simulink library "myLibrary"  (R2023b)
settings: Solver=VariableStepAuto  StartTime=0.0  StopTime=10.0  RelTol=1e-3
undefined symbols (not defined in the file): Cac_n1, ctrl1, Da, delta_slk, Discrete, dtha, ee_sli_rtmsupport, FA, gcbh, Ha, Ini, init_DCline, init_IPC, init_line, init_load, init_SG, init_shunt, init_TH, init_trafo, init_user, init_VSC, initMachineBlocks, Ka, Lf, Llkd_pu, Llkq1_pu, magnitude, NET, P, plots_step, q0, Rac_n1, Radd, Rkd_pu, Rkq1_pu, Rload_add, sim_config, sps_rtmsupport, spsSteamTurbineModel, T_DC_NET, T_global, T_IPC, T_load, T_NET, T_SG, T_shunt, T_STATCOM, T_TH, T_trafo, T_user, T_VSC, Ts, tstep, Udiff_a, V1
libraries: spsSeriesRLCBranchLib x120, eeGeneralControl x83, $bdroot x78, spsCurrentMeasurementLib x53, spsParallelRLCBranchLib x39, spsVoltageMeasurementLib x37, spsControlledVoltageSourceLib x30, simulink x29, spsFirstOrderFilterLib x18, spsMeasurementModel x13, spsThreePhaseVIMeasurementLib x5, dspsigops x4
(part 4 of 16)

== system myLibrary/SG_step ==
  Add : Sum  Inputs=-+
  Add1 : Sum
  Add2 : Sum  Inputs=+-
  Bus Selector : BusSelector  OutputSignals="Mechanical.Electromagnetic torque  Te (pu),dq0 components.Stator current  iq (pu),dq0 components.Stator current  id (pu),dq0 components.Field current  ifd (pu),dq0 components.Damper winding current  ikd (pu),dq0 components.Damper winding current  ikq1 (pu),dq0 components.Damper winding current  ikq2 (pu),dq0 components.Stator voltage  vq (pu),dq0 components.Stator voltage  vd (pu),Mechanical.Rotor angle deviation  d_theta (rad),Mechanical.Rotor speed  wm (pu),Mechanical.Rotor mechanical angle  theta (deg),Load angle   delta  (deg)"
  Constant4 : Constant  Value=[2/3 1/3; -1/3 1/3 ; -1/3 -2/3]
  Constant_pi1 : Constant  Value=pi/2
  Constant_pi2 : Constant  Value=-pi/2
  Current Measurement3 : spsCurrentMeasurementLib/Current Measurement  PhasorSimulation=off  OutputType=Complex  PSBequivalent=0
  Demux4 : Demux  Outputs=3
  Display : Display
  Display1 : Display
  Exciter : Subsystem
  Gain : Gain  Gain=T_SG.wb
  Gain1 : Gain  Gain=pi/180
  Gain2 : Gain  Gain=1/T_SG.Lmd_pu
  Gain3 : Gain  Gain=pi/180
  Governor-Turbine : Subsystem
  Integrator : Integrator
  Mux4 : Mux  Inputs=2
  PLL (3ph) : spsPLL3phLib/PLL (3ph)  Fmin=45  Par_Init=[0, 50]  ParK=[180, 3200, 1]  TcD=1e-4  MaxRateChangeFreq=12  FilterCutOffFreq=25  Ts=0  AGC=on
  PLL (3ph)1 : spsPLL3phLib/PLL (3ph)  Fmin=45  Par_Init=[initSG.theta_in, 50]  ParK=[180, 3200, 1]  TcD=1e-4  MaxRateChangeFreq=12  FilterCutOffFreq=25  Ts=0  AGC=on
  Pm : Step  Time=tstep_P  Before=initSG.Pm  After=initSG.Pm*(1+sim_config.DR)  SampleTime=1e-4
  SM1 : spsSynchronousMachinepuFundamentalLib/Synchronous Machine pu Fundamental  PresetModel=No  MechanicalLoad=Mechanical power Pm  ShowDetailedParameters=on  RotorType=Round  Units=per unit fundamental parameters  MeasurementBus=off  NominalParameters=initMachineBlocks{SGnum,1}  Stator=initMachineBlocks{SGnum,2}  Field=initMachineBlocks{SGnum,3}  Dampers2=initMachineBlocks{SGnum,4}  Dampers1="[ Rkd_pu   Llkd_pu  Rkq1_pu  Llkq1_pu]"  Mechanical=initMachineBlocks{SGnum,5}  PolePairs=1  InitialConditions=initMachineBlocks{SGnum,6}  SetSaturation=off  Saturation=[0.6404,0.7127,0.8441,0.9214,0.9956,1.082,1.19,1.316,1.457;0.7,0.7698,0.8872,0.9466,0.9969,1.046,1.1,1.151,1.201]  LoadFlowParameters=[1 5.55 0 0 0]  TsPowergui=0  TsBlock=-1  IterativeModel=Trapezoidal non iterative  IterativeDiscreteModel=Trapezoidal non iterative  BusType=PV  Pref=5.55  Qref=0  Qmin=-Inf  Qmax=Inf  PLF=0  QLF=0
  Scope{,1..2,4,6,10} (6 alike) : Scope
  Scope3 : Scope  NumInputPorts=3
  Scope5 : Scope  NumInputPorts=2
  Scope7 : Scope  NumInputPorts=2
  Series RLC Branch1 : spsSeriesRLCBranchLib/Series RLC Branch  LConnTagsString=__new0  RConnTagsString=__new0  BranchType=RL  Resistance=T_SG.Rtr*T_SG.Zbpu_l2g  Inductance=T_SG.Ltr*T_SG.Zbpu_l2g  SetiL0=off  InitialCurrent=initSG.Itr  Capacitance=P.C  Setx0=on  InitialVoltage=P.C  Measurements=None
  Series RLC Branch2 : PMComponent  DialogController=POWERSYS.PowerSysDialog  LoadFcn=sps_rtmsupport('LoadFcn',gcbh);  StartFcn=sps_rtmsupport('StartFcn',gcbh);  StopFcn=sps_rtmsupport('StopFcn',gcbh);  PhysicalDomain=powersysdomain  LeftPortType=p1  RightPortType=p1  LConnTagsString=__new0  RConnTagsString=__new0  mask(Series RLC Branch){BranchType=RL, Resistance=T_SG.Rtr*T_SG.Zbpu_l2g, Inductance=T_SG.Ltr*T_SG.Zbpu_l2g, SetiL0=off, InitialCurrent=initSG.Itr, Capacitance=P.C, Setx0=on, InitialVoltage=P.C, Measurements=None}
      mask prompts: BranchType "Branch type:"; Resistance "Resistance (Ohms):"; Inductance "Inductance (H):"; SetiL0 "Set the initial inductor current"; InitialCurrent "Inductor initial current (A):"; Capacitance "Capacitance (F):"; Setx0 "Set the initial capacitor voltage"; InitialVoltage "Capacitor initial voltage (V):"
      mask help:
      | Implements a series branch of RLC elements.
      | Use the 'Branch type' parameter to add or remove elements from the branch.
      mask init:
      | [s1,s2,s3,s4,r1,r2,l1,l2,c1,c2,c3,c4] = powericon('Series RLC Branch',Resistance,Inductance,Capacitance,BranchType);
      | powericon('RLCCback',gcb)
      | power_initmask();
      settings: LibrarySourceBlock=spsSeriesRLCBranchLib/Series RLC Branch  CopyFcn=sps_rtmsupport('CopyFcn',gcbh);  DeleteFcn=sps_rtmsupport('DeleteFcn',gcbh);  UndoDeleteFcn=sps_rtmsupport('UndoDeleteFcn',gcbh);  ModelCloseFcn=sps_rtmsupport('ModelCloseFcn',gcbh);  PreSaveFcn=sps_rtmsupport('PreSaveFcn',gcbh);  PostSaveFcn=sps_rtmsupport('PostSaveFcn',gcbh);  NameChangeFcn=sps_rtmsupport('NameChangeFcn',gcbh);  PreCopyFcn=sps_rtmsupport('PreCopyFcn',gcbh);  OpenFcn=sps_rtmsupport('OpenFcn',gcbh, [1 4 7 9]);  CloseFcn=sps_rtmsupport('CloseFcn',gcbh);  PreDeleteFcn=sps_rtmsupport('PreDeleteFcn',gcbh);
      mask Help: helpview(psbhelp);
      mask TypeOptions BranchType: RLC | R | L | C | RL | RC | LC | Open circuit
      mask Callback BranchType: powericon('RLCCback',gcb)
      mask Callback Resistance: powericon('RLCCback',gcb)
      mask Callback Inductance: powericon('RLCCback',gcb)
      mask Callback SetiL0: powericon('RLCCback',gcb)
      mask Callback Capacitance: powericon('RLCCback',gcb)
      mask Callback Setx0: powericon('RLCCback',gcb)
      mask TypeOptions Measurements: None | Branch voltage | Branch current | Branch voltage and current
      mask Display:
      | plot(s1,s2,s3,s4,r1,r2*1.5,l1,l2*1.5,c1,c2*1.5,c3,c4*1.5)
      | color('red')
      | port_label('LConn',1,'+')
  Series RLC Branch3 : PMComponent  DialogController=POWERSYS.PowerSysDialog  LoadFcn=sps_rtmsupport('LoadFcn',gcbh);  StartFcn=sps_rtmsupport('StartFcn',gcbh);  StopFcn=sps_rtmsupport('StopFcn',gcbh);  PhysicalDomain=powersysdomain  LeftPortType=p1  RightPortType=p1  LConnTagsString=__new0  RConnTagsString=__new0  mask(Series RLC Branch){BranchType=RL, Resistance=T_SG.Rtr*T_SG.Zbpu_l2g, Inductance=T_SG.Ltr*T_SG.Zbpu_l2g, SetiL0=off, InitialCurrent=initSG.Itr, Capacitance=P.C, Setx0=on, InitialVoltage=P.C, Measurements=None}
      mask prompts: BranchType "Branch type:"; Resistance "Resistance (Ohms):"; Inductance "Inductance (H):"; SetiL0 "Set the initial inductor current"; InitialCurrent "Inductor initial current (A):"; Capacitance "Capacitance (F):"; Setx0 "Set the initial capacitor voltage"; InitialVoltage "Capacitor initial voltage (V):"
      mask help:
      | Implements a series branch of RLC elements.
      | Use the 'Branch type' parameter to add or remove elements from the branch.
      mask init:
      | [s1,s2,s3,s4,r1,r2,l1,l2,c1,c2,c3,c4] = powericon('Series RLC Branch',Resistance,Inductance,Capacitance,BranchType);
      | powericon('RLCCback',gcb)
      | power_initmask();
      settings: LibrarySourceBlock=spsSeriesRLCBranchLib/Series RLC Branch  CopyFcn=sps_rtmsupport('CopyFcn',gcbh);  DeleteFcn=sps_rtmsupport('DeleteFcn',gcbh);  UndoDeleteFcn=sps_rtmsupport('UndoDeleteFcn',gcbh);  ModelCloseFcn=sps_rtmsupport('ModelCloseFcn',gcbh);  PreSaveFcn=sps_rtmsupport('PreSaveFcn',gcbh);  PostSaveFcn=sps_rtmsupport('PostSaveFcn',gcbh);  NameChangeFcn=sps_rtmsupport('NameChangeFcn',gcbh);  PreCopyFcn=sps_rtmsupport('PreCopyFcn',gcbh);  OpenFcn=sps_rtmsupport('OpenFcn',gcbh, [1 4 7 9]);  CloseFcn=sps_rtmsupport('CloseFcn',gcbh);  PreDeleteFcn=sps_rtmsupport('PreDeleteFcn',gcbh);
      mask Help: helpview(psbhelp);
      mask TypeOptions BranchType: RLC | R | L | C | RL | RC | LC | Open circuit
      mask Callback BranchType: powericon('RLCCback',gcb)
      mask Callback Resistance: powericon('RLCCback',gcb)
      mask Callback Inductance: powericon('RLCCback',gcb)
      mask Callback SetiL0: powericon('RLCCback',gcb)
      mask Callback Capacitance: powericon('RLCCback',gcb)
      mask Callback Setx0: powericon('RLCCback',gcb)
      mask TypeOptions Measurements: None | Branch voltage | Branch current | Branch voltage and current
      mask Display:
      | plot(s1,s2,s3,s4,r1,r2*1.5,l1,l2*1.5,c1,c2*1.5,c3,c4*1.5)
      | color('red')
      | port_label('LConn',1,'+')
  Sum : Sum  Inputs=++++
  Te : Scope
  Three-Phase Series RLC Branch4 : spsThreePhaseSeriesRLCBranchLib/Three-Phase Series RLC Branch  LConnTagsString=A|B|C  RConnTagsString=A|B|C  BranchType=R  Resistance=T_SG.Rsnb*T_SG.Zbpu_l2g  Inductance=NET.L1_2/2  Capacitance=1/0.0528/(2*pi*50)  Measurements=None
  Three-Phase V-I Measurement : spsThreePhaseVIMeasurementLib/Three-Phase V-I Measurement  VoltageMeasurement=phase-to-phase  SetLabelV=off  LabelV=Vpcc  Vpu=off  VpuLL=off  CurrentMeasurement=no  SetLabelI=off  LabelI=Iabc  Ipu=off  Pbase=100e6  Vbase=500e3  OutputType=Complex  PhasorSimulation=off  PSBequivalent=0
  Three-Phase V-I Measurement1 : spsThreePhaseVIMeasurementLib/Three-Phase V-I Measurement  VoltageMeasurement=phase-to-phase  SetLabelV=off  LabelV=Vtr  Vpu=off  VpuLL=off  CurrentMeasurement=no  SetLabelI=off  LabelI=Iabc  Ipu=off  Pbase=100e6  Vbase=500e3  OutputType=Complex  PhasorSimulation=off  PSBequivalent=0
  Unwrap : dspsigops/Unwrap  tol=pi  InputProcessing=Columns as channels (frame based)  running=off
  Unwrap1 : dspsigops/Unwrap  tol=pi  InputProcessing=Columns as channels (frame based)  running=off
  Unwrap2 : dspsigops/Unwrap  tol=pi  InputProcessing=Columns as channels (frame based)  running=off
  "Vector magnitude " : Subsystem
  Vf : Constant  Value=initSG.Vf
  deg2rad : Gain  Gain=pi/180
  isqd : Scope  NumInputPorts=2
  mtx4 : Product  Multiplication=Matrix(*)
  qd3 : $bdroot/qd transform  SystemSampleTime=-1  VariantActivationTime=update diagram  AllowFlexibleInterface=on  Latency=0  AutoFrameSizeCalculation=off
  v_ref : Step  Time=tstep_V  Before=initSG.Vref  After=initSG.Vref*(1+sim_config.DR)  SampleTime=1e-4
  vqd : Scope  NumInputPorts=3
  A : PMIOPort  Side=Right
  B : PMIOPort  Port=2  Side=Right
  C : PMIOPort  Port=3  Side=Right
  tag scope: V_fn_pcc=global, theta_SG1=global, w_SG1=global
  wires:
  Three-Phase V-I Measurement1/1 -> [Vtr]
  Three-Phase V-I Measurement/1 -> [Vpcc]
  Bus Selector/10 -> [d_theta], Add1/1, Scope/1  "<Rotor angle deviation  d_theta (rad)>"
  Bus Selector/7 -> [ikq2]  "<Damper winding current  ikq2 (pu)>"
  [Vtr] -> PLL (3ph)/1
  Gain2/1 -> Scope1/1, [ifd]
  Bus Selector/5 -> [ikd]  "<Damper winding current  ikd (pu)>"
  Bus Selector/3 -> isqd/2, [isd]  "<Stator current  id (pu)>"
  Bus Selector/11 -> [we], Gain/1  "<Rotor speed  wm (pu)>"
  Bus Selector/6 -> [ikq1]  "<Damper winding current  ikq1 (pu)>"
  [Vpcc] -> PLL (3ph)1/1
  Bus Selector/4 -> Gain2/1  "<Field current  ifd (pu)>"
  Bus Selector/8 -> "Vector magnitude "/1(Vq), vqd/1, [vq]  "<Stator voltage  vq (pu)>"
  Bus Selector/1 -> Te/1, [Te]  "<Electromagnetic torque  Te (pu)>"
  Bus Selector/9 -> "Vector magnitude "/2(Vd), vqd/2, [vd]  "<Stator voltage  vd (pu)>"
  Gain/1 -> Scope6/1, [w_SG1], Integrator/1
  Current Measurement3/1 -> Scope2/1  "a"
  "Vector magnitude "/1(V) -> vqd/3  "V"
  Unwrap1/1 -> Add/1
  SM1/1 -> Bus Selector/1
  Bus Selector/13 -> [delta], Gain1/1, Gain3/1  "<Load angle   delta  (deg)>"
  Bus Selector/12 -> deg2rad/1, [theta]  "<Rotor mechanical angle  theta (deg)>"
  Bus Selector/2 -> isqd/1, [isq]  "<Stator current  iq (pu)>"
  Add/1 -> Scope4/1, Sum/4  "theta_in"
  Integrator/1 -> Sum/2
  PLL (3ph)1/2 -> Unwrap/1
  PLL (3ph)/2 -> Unwrap1/1
  Unwrap/1 -> Add/2
  Constant_pi1/1 -> Add1/2
  Add1/1 -> Scope5/1  "d_theta"
  Gain3/1 -> Scope5/2  "load_angle"
  Gain1/1 -> Sum/3
  Constant_pi2/1 -> Sum/1
  Governor-Turbine/1(Pm) -> SM1/1
  [we] -> Governor-Turbine/2(wm)  "wm"
  Pm/1 -> Governor-Turbine/1(Pref)
  [d_theta] -> Governor-Turbine/3(d_theta)
  deg2rad/1 -> Unwrap2/1
  Unwrap2/1 -> Add2/2, Scope3/3, [theta_SG1]  "THETA MATLAB"
  [we] -> Exciter/4(Vsi1)
  [vd] -> Exciter/3(Vd)
  [ifd] -> Exciter/6(Ifd_pu)
  [Te] -> Exciter/5(Vsi2)
  Vf/1 -> Exciter/7(Efd0_pu)
  v_ref/1 -> Exciter/1(V_REF)
  Exciter/1(Out1) -> SM1/2
  [vq] -> Exciter/2(Vq)
  Sum/1 -> Scope3/2, Add2/1  "OUR CALC"
  Add2/1 -> Scope3/1  "RESTA"
  qd3/1 -> Display/1, Scope7/1
  Demux4/1 -> Mux4/1
  [Vpcc] -> Demux4/1
  [V_fn_pcc] -> qd3/1
  Constant4/1 -> mtx4/1
  Demux4/2 -> Mux4/2
  Mux4/1 -> mtx4/2
  mtx4/1 -> [V_fn_pcc], Scope10/1
  qd3/2 -> Display1/1, Scope7/2
  [theta_SG1] -> qd3/2
  connections:
  Three-Phase V-I Measurement/LConn3 -- SM1/RConn3
  SM1/RConn2 -- Three-Phase V-I Measurement/LConn2
  Three-Phase V-I Measurement/LConn1 -- SM1/RConn1
  B/RConn1 -- Three-Phase V-I Measurement1/RConn2
  Series RLC Branch3/RConn1 -- Three-Phase V-I Measurement1/LConn3
  Series RLC Branch1/RConn1 -- Three-Phase V-I Measurement1/LConn1
  Current Measurement3/RConn1 -- Three-Phase Series RLC Branch4/RConn1
  A/RConn1 -- Three-Phase V-I Measurement1/RConn1
  C/RConn1 -- Three-Phase V-I Measurement1/RConn3
  Series RLC Branch2/RConn1 -- Three-Phase V-I Measurement1/LConn2
  Three-Phase V-I Measurement/RConn1 -- Series RLC Branch1/LConn1 -- Current Measurement3/LConn1
  Three-Phase V-I Measurement/RConn3 -- Series RLC Branch3/LConn1 -- Three-Phase Series RLC Branch4/RConn3
  Three-Phase Series RLC Branch4/LConn3 -- Three-Phase Series RLC Branch4/LConn2 -- Three-Phase Series RLC Branch4/LConn1
  Three-Phase V-I Measurement/RConn2 -- Series RLC Branch2/LConn1 -- Three-Phase Series RLC Branch4/RConn2

== system myLibrary/STATCOM ==
  Constant5 : Constant  Value=[ 2/3 1/3; -1/3 1/3 ; -1/3 -2/3]
  Control : Subsystem
      settings: PortSchema="{\"entries\":[{\"content\":{\"sides\":[{\"content\":{},\"type\":\"ConnectorPlacement.EquallySpacedRectSide\",\"uuid\":\"681c0b5f-022d-4b6d-8fe2-73940743a76e\"},{\"content\":{\"side\":\"RIGHT\"},\"type\":\"ConnectorPlacement.EquallySpacedRectSide\",\"uuid\":\"e9b400c8-e13f-4caf-91a1-f348979675fd\"},{\"content\":{\"connectorIds\":[\"In1\",\"Out1\",\"Out2\"],\"side\":\"TOP\"},\"type\":\"ConnectorPlacement.EquallySpacedRectSide\",\"uuid\":\"348007cb-ce67-4c45-ad7b-36ba89db6185\"},{\"content\":{\"connectorIds\":[\"In2\",\"In3\",\"In4\"],\"side\":\"BOTTOM\"},\"type\":\"ConnectorPlacement.EquallySpacedRectSide\",\"uuid\":\"fd6a847a-5d69-44cd-a0d1-495126761350\"}]},\"type\":\"ConnectorPlacement.EquallySpacedConnector\",\"uuid\":\"d16b8cae-5ced-4c76-a87e-983e154fb48f\"}],\"packageUris\":[\"http://schema.mathworks.com/mf0/Connector/R2020b\"],\"version\":\"1.0\"}"
  Current Measurement20 : spsCurrentMeasurementLib/Current Measurement  PhasorSimulation=off  OutputType=Complex  PSBequivalent=0
  Current Measurement21 : spsCurrentMeasurementLib/Current Measurement  PhasorSimulation=off  OutputType=Complex  PSBequivalent=0
  Current Measurement25 : spsCurrentMeasurementLib/Current Measurement  PhasorSimulation=off  OutputType=Complex  PSBequivalent=0
  Electrical : Subsystem
  Ig_l2g : Gain  Gain=1/T_VSC.Sbpu_l2g
  Is_l2g : Gain  Gain=1/T_VSC.Sbpu_l2g
  Mux10 : Mux  Inputs=2
  Mux4 : Mux  Inputs=3
  Product4 : Product  Multiplication=Matrix(*)
  Scope : Scope  NumInputPorts=3
  Series RLC Branch1 : spsSeriesRLCBranchLib/Series RLC Branch  LConnTagsString=__new0  RConnTagsString=__new0  BranchType=RL  Resistance=initVSC.Rtr  Inductance=initVSC.Ltr  SetiL0=off  InitialCurrent=initVSC.Iga  Capacitance=P.C  Setx0=on  InitialVoltage=P.C  Measurements=None
  Series RLC Branch10 : spsSeriesRLCBranchLib/Series RLC Branch  LConnTagsString=__new0  RConnTagsString=__new0  BranchType=R  Resistance=initVSC.Rac  Inductance=Lf  SetiL0=off  InitialCurrent=0  Capacitance=Cac_n1  Setx0=on  InitialVoltage=vcini_n1  Measurements=None
  Series RLC Branch2 : spsSeriesRLCBranchLib/Series RLC Branch  LConnTagsString=__new0  RConnTagsString=__new0  BranchType=RL  Resistance=initVSC.Rtr  Inductance=initVSC.Ltr  SetiL0=on  InitialCurrent=initVSC.Igb  Capacitance=P.C  Setx0=on  InitialVoltage=P.C  Measurements=None
  Series RLC Branch3 : spsSeriesRLCBranchLib/Series RLC Branch  LConnTagsString=__new0  RConnTagsString=__new0  BranchType=RL  Resistance=initVSC.Rtr  Inductance=initVSC.Ltr  SetiL0=on  InitialCurrent=initVSC.Igc  Capacitance=P.C  Setx0=on  InitialVoltage=P.C  Measurements=None
  Series RLC Branch4 : spsSeriesRLCBranchLib/Series RLC Branch  LConnTagsString=__new0  RConnTagsString=__new0  BranchType=C  Resistance=Rac_n1  Inductance=Lf  SetiL0=off  InitialCurrent=0  Capacitance=initVSC.Cac  Setx0=on  InitialVoltage=initVSC.Ucap_b  Measurements=None
  Series RLC Branch5 : spsSeriesRLCBranchLib/Series RLC Branch  LConnTagsString=__new0  RConnTagsString=__new0  BranchType=C  Resistance=Rac_n1  Inductance=Lf  SetiL0=off  InitialCurrent=0  Capacitance=initVSC.Cac  Setx0=on  InitialVoltage=initVSC.Ucap_a  Measurements=None
  Series RLC Branch6 : spsSeriesRLCBranchLib/Series RLC Branch  LConnTagsString=__new0  RConnTagsString=__new0  BranchType=R  Resistance=initVSC.Rac  Inductance=Lf  SetiL0=off  InitialCurrent=0  Capacitance=Cac_n1  Setx0=on  InitialVoltage=vcini_n1  Measurements=None
  Series RLC Branch8 : spsSeriesRLCBranchLib/Series RLC Branch  LConnTagsString=__new0  RConnTagsString=__new0  BranchType=R  Resistance=initVSC.Rac  Inductance=Lf  SetiL0=off  InitialCurrent=0  Capacitance=Cac_n1  Setx0=on  InitialVoltage=vcini_n1  Measurements=None
  Series RLC Branch9 : spsSeriesRLCBranchLib/Series RLC Branch  LConnTagsString=__new0  RConnTagsString=__new0  BranchType=C  Resistance=Rac_n1  Inductance=Lf  SetiL0=off  InitialCurrent=0  Capacitance=initVSC.Cac  Setx0=on  InitialVoltage=initVSC.Ucap_c  Measurements=None
  U_g2l : Gain
  Vdiff_l2g : Gain
  Voltage Measurement{,1..4} (5 alike) : spsVoltageMeasurementLib/Voltage Measurement  PhasorSimulation=off  OutputType=Complex  PSBequivalent=0
  VA : PMIOPort  Side=Right
  VB : PMIOPort  Port=2  Side=Right
  VC : PMIOPort  Port=3  Side=Right
  wires:
  Voltage Measurement1/1 -> Mux10/2
  Constant5/1 -> Product4/1
  Mux10/1 -> Product4/2
  Voltage Measurement/1 -> Mux10/1
  Product4/1 -> U_g2l/1
  Control/1(Vdiff_abc) -> Vdiff_l2g/1
  Electrical/2(Is) -> Is_l2g/1
  Vdiff_l2g/1 -> Electrical/2(vdiff)
  Is_l2g/1 -> Control/3(Iss)
  U_g2l/1 -> Control/2(U)
  Current Measurement20/1 -> Mux4/2
  Current Measurement21/1 -> Mux4/1
  Mux4/1 -> Ig_l2g/1
  Current Measurement25/1 -> Mux4/3
  Ig_l2g/1 -> Control/1(ig_abc)
  Voltage Measurement3/1 -> Scope/2
  Voltage Measurement2/1 -> Scope/1
  Voltage Measurement4/1 -> Scope/3
  Control/2(Pac) -> Electrical/1(Pac)
  Electrical/1(Vdc) -> Control/4(Vdc)
  connections:
  VB/RConn1 -- Current Measurement20/RConn1
  Series RLC Branch1/LConn1 -- Series RLC Branch5/LConn1 -- Voltage Measurement2/LConn1 -- Voltage Measurement/LConn1 -- Electrical/LConn1
  Voltage Measurement1/LConn2 -- Series RLC Branch9/LConn1 -- Voltage Measurement4/LConn1 -- Series RLC Branch3/LConn1 -- Electrical/LConn3
  VA/RConn1 -- Current Measurement21/RConn1
  Voltage Measurement1/LConn1 -- Series RLC Branch4/LConn1 -- Voltage Measurement3/LConn1 -- Series RLC Branch2/LConn1 -- Voltage Measurement/LConn2 -- Electrical/LConn2
  Current Measurement25/RConn1 -- VC/RConn1
  Series RLC Branch1/RConn1 -- Current Measurement21/LConn1
  Series RLC Branch2/RConn1 -- Current Measurement20/LConn1
  Series RLC Branch3/RConn1 -- Current Measurement25/LConn1
  Voltage Measurement2/LConn2 -- Series RLC Branch6/LConn1 -- Series RLC Branch5/RConn1
  Voltage Measurement3/LConn2 -- Series RLC Branch4/RConn1 -- Series RLC Branch8/LConn1
  Voltage Measurement4/LConn2 -- Series RLC Branch10/LConn1 -- Series RLC Branch9/RConn1
  Series RLC Branch10/RConn1 -- Series RLC Branch8/RConn1 -- Series RLC Branch6/RConn1

== system myLibrary/TH ==
  note: Grid Thevenin
  Series RLC Branch : spsSeriesRLCBranchLib/Series RLC Branch  LConnTagsString=__new0  RConnTagsString=__new0  BranchType=RL  Resistance=T.R  Inductance=T.L  SetiL0=off  InitialCurrent=ini.Itha  Capacitance=1e-6  Setx0=off  InitialVoltage=0  Measurements=None
  Series RLC Branch1 : spsSeriesRLCBranchLib/Series RLC Branch  LConnTagsString=__new0  RConnTagsString=__new0  BranchType=RL  Resistance=T.R  Inductance=T.L  SetiL0=on  InitialCurrent=ini.Ithb  Capacitance=1e-6  Setx0=off  InitialVoltage=0  Measurements=None
  Series RLC Branch2 : spsSeriesRLCBranchLib/Series RLC Branch  LConnTagsString=__new0  RConnTagsString=__new0  BranchType=RL  Resistance=T.R  Inductance=T.L  SetiL0=on  InitialCurrent=ini.Ithc  Capacitance=1e-6  Setx0=off  InitialVoltage=0  Measurements=None
  Three-Phase Source : spsThreePhaseSourceLib/Three-Phase Source  InternalConnection=Y  VoltagePhases=off  Voltage=ini.Vmag  PhaseAngle=ini.angle*180/pi  Voltage_phases=[25e3 25e3 25e3]/sqrt(3)  PhaseAngles_phases=[0 -120 +120]  Frequency="T_global{T_global.Area == T.Area,\"fb\"}"  NonIdealSource=off  SpecifyImpedance=off  Resistance=0.8929  Inductance=16.58e-3  ShortCircuitLevel=100e6  BaseVoltage=25e3  XRratio=7  BusType=swing  Pref=10e3  Qref=0  Prefabc=[10e3, 10e3, 10e3]  Qrefabc=[0, 0, 0]  Qmin=-inf  Qmax=inf
  A : PMIOPort  Side=Right
  B : PMIOPort  Port=2  Side=Right
  C : PMIOPort  Port=3  Side=Right
  connections:
  Series RLC Branch1/LConn1 -- Three-Phase Source/RConn2
  Series RLC Branch/LConn1 -- Three-Phase Source/RConn1
  A/RConn1 -- Series RLC Branch/RConn1
  B/RConn1 -- Series RLC Branch1/RConn1
  Series RLC Branch2/LConn1 -- Three-Phase Source/RConn3
  C/RConn1 -- Series RLC Branch2/RConn1

== system myLibrary/TH_step ==
  note: Grid Thevenin
  Constant1 : Constant  Value="2*pi*T_global{T_global.Area == T.Area,\"fb\"}"
  Constant2 : Constant  Value=2*pi/3
  Controlled Voltage Source : spsControlledVoltageSourceLib/Controlled Voltage Source  Initialize=on  Source_Type=AC  Amplitude=ini.Vmag/sqrt(3)*sqrt(2)  Phase=ini.angle*180/pi  Frequency=T_global.f_Hz(T.Area)  Measurements=None
  Controlled Voltage Source3 : spsControlledVoltageSourceLib/Controlled Voltage Source  Initialize=on  Source_Type=AC  Amplitude=ini.Vmag/sqrt(3)*sqrt(2)  Phase=ini.angle*180/pi-120  Frequency=T_global.f_Hz(T.Area)  Measurements=None
  Controlled Voltage Source4 : spsControlledVoltageSourceLib/Controlled Voltage Source  Initialize=on  Source_Type=AC  Amplitude=ini.Vmag/sqrt(3)*sqrt(2)  Phase=ini.angle*180/pi+120  Frequency=T_global.f_Hz(T.Area)  Measurements=None
  Ground : spsGroundLib/Ground  LConnTagsString=a
  Integrator : Integrator  InitialCondition=ini.angle
  Product : Product
  Product1 : Product
  Product2 : Product
  Series RLC Branch : spsSeriesRLCBranchLib/Series RLC Branch  LConnTagsString=__new0  RConnTagsString=__new0  BranchType=RL  Resistance=T.R  Inductance=T.L  SetiL0=on  InitialCurrent=ini.Itha  Capacitance=1e-6  Setx0=off  InitialVoltage=0  Measurements=None
  Series RLC Branch1 : spsSeriesRLCBranchLib/Series RLC Branch  LConnTagsString=__new0  RConnTagsString=__new0  BranchType=RL  Resistance=T.R  Inductance=T.L  SetiL0=on  InitialCurrent=ini.Ithb  Capacitance=1e-6  Setx0=off  InitialVoltage=0  Measurements=None
  Series RLC Branch2 : spsSeriesRLCBranchLib/Series RLC Branch  LConnTagsString=__new0  RConnTagsString=__new0  BranchType=RL  Resistance=T.R  Inductance=T.L  SetiL0=on  InitialCurrent=ini.Ithc  Capacitance=1e-6  Setx0=off  InitialVoltage=0  Measurements=None
  Sin : Trigonometry
  Sin1 : Trigonometry
  Sin2 : Trigonometry
  Step : Step  Time=tstep  Before=ini.Vmag/sqrt(3)*sqrt(2)  After=V1/sqrt(3)*sqrt(2)  SampleTime=1e-4
  Sum : Sum  Inputs=+-
  Sum1 : Sum
  A : PMIOPort  Side=Right
  B : PMIOPort  Port=2  Side=Right
  C : PMIOPort  Port=3  Side=Right
  wires:
  Sum1/1 -> Sin2/1
  Sin/1 -> Product/1
  Product1/1 -> Controlled Voltage Source3/1
  Product/1 -> Controlled Voltage Source/1
  Sum/1 -> Sin1/1
  Sin1/1 -> Product1/1
  Step/1 -> Product2/2, Product1/2, Product/2
  Sin2/1 -> Product2/1
  Product2/1 -> Controlled Voltage Source4/1
  Constant1/1 -> Integrator/1
  Constant2/1 -> Sum1/2, Sum/2
  Integrator/1 -> Sum/1, Sum1/1, Sin/1
  connections:
  Series RLC Branch1/LConn1 -- Controlled Voltage Source3/RConn1
  Series RLC Branch/LConn1 -- Controlled Voltage Source/RConn1
  Series RLC Branch1/RConn1 -- B/RConn1
  A/RConn1 -- Series RLC Branch/RConn1
  Controlled Voltage Source4/RConn1 -- Series RLC Branch2/LConn1
  C/RConn1 -- Series RLC Branch2/RConn1
  Controlled Voltage Source/LConn1 -- Controlled Voltage Source4/LConn1 -- Ground/LConn1 -- Controlled Voltage Source3/LConn1

== system myLibrary/Trafo ==
  Series RLC Branch1 : spsSeriesRLCBranchLib/Series RLC Branch  LConnTagsString=__new0  RConnTagsString=__new0  BranchType=RL  Resistance=T.R  Inductance=T.L  SetiL0=on  InitialCurrent=ini.Ia  Capacitance=P.C  Setx0=on  InitialVoltage=P.C  Measurements=None
  Series RLC Branch2 : spsSeriesRLCBranchLib/Series RLC Branch  LConnTagsString=__new0  RConnTagsString=__new0  BranchType=RL  Resistance=T.R  Inductance=T.L  SetiL0=on  InitialCurrent=ini.Ib  Capacitance=P.C  Setx0=on  InitialVoltage=P.C  Measurements=None
  Series RLC Branch3 : spsSeriesRLCBranchLib/Series RLC Branch  LConnTagsString=__new0  RConnTagsString=__new0  BranchType=RL  Resistance=T.R  Inductance=T.L  SetiL0=on  InitialCurrent=ini.Ic  Capacitance=P.C  Setx0=on  InitialVoltage=P.C  Measurements=None
  A1 : PMIOPort  Side=Left
  B1 : PMIOPort  Port=2  Side=Left
  C1 : PMIOPort  Port=3  Side=Left
  A2 : PMIOPort  Port=4  Side=Right
  B2 : PMIOPort  Port=5  Side=Right
  C2 : PMIOPort  Port=6  Side=Right
  connections:
  Series RLC Branch1/RConn1 -- A2/RConn1
  Series RLC Branch2/RConn1 -- B2/RConn1
  Series RLC Branch3/RConn1 -- C2/RConn1
  Series RLC Branch2/LConn1 -- B1/RConn1
  Series RLC Branch1/LConn1 -- A1/RConn1
  Series RLC Branch3/LConn1 -- C1/RConn1

== system myLibrary/User-Linear ==
  note: Use the state-space system
  Constant : Constant  Value=0
  Constant1 : Constant  Value=inituser.ig_q0
  Constant2 : Constant  Value=inituser.ig_d0
  Constant3 : Constant  Value=inituser.vg_q0
  Constant4 : Constant  Value=inituser.vg_d0
  Constant5 : Constant  Value=[ 2/3 1/3; -1/3 1/3 ; -1/3 -2/3]
  Constant8 : Constant  Value=0
  Controlled Current Source : spsControlledCurrentSourceLib/Controlled Current Source  Initialize=on  Source_Type=AC  Amplitude=abs(inituser.Igabc)*sqrt(2)  Phase=angle(inituser.Igabc)*180/pi  Frequency=T_user.fn(num)  Measurements=None
  Controlled Current Source1 : spsControlledCurrentSourceLib/Controlled Current Source  Initialize=on  Source_Type=AC  Amplitude=abs(inituser.Igabc)*sqrt(2)  Phase=angle(inituser.Igabc)*180/pi-120  Frequency=T_user.fn(num)  Measurements=None
  Current Measurement : spsCurrentMeasurementLib/Current Measurement  PhasorSimulation=off  OutputType=Complex  PSBequivalent=0
  Current Measurement1 : Subsystem  DialogController=POWERSYS.PowerSysDialog  LoadFcn=sps_rtmsupport('LoadFcn',gcbh);  StartFcn=sps_rtmsupport('StartFcn',gcbh);  StopFcn=sps_rtmsupport('StopFcn',gcbh);  mask(Current Measurement){PhasorSimulation=off, OutputType=Complex, PSBequivalent=0}
      mask prompts: PhasorSimulation "Phasor simulation"; OutputType "Output signal :"; PSBequivalent "Equivalent circuit"
      mask help: Ideal current measurement. The Output signal parameter is disabled when the block is not used in a phasor simulation. The phasor simulation is activated by a Powergui block placed in the model.
      mask init: same as myLibrary/HVDC_line/Current Measurement1
      settings: LibrarySourceBlock=sps_lib/Sensors and Measurements/Current Measurement  CopyFcn=sps_rtmsupport('CopyFcn',gcbh); powericon('psbloadfunction',gcb,'Measurement Block','UpdateGotoTag');  DeleteFcn=sps_rtmsupport('DeleteFcn',gcbh);  UndoDeleteFcn=sps_rtmsupport('UndoDeleteFcn',gcbh);  ModelCloseFcn=sps_rtmsupport('ModelCloseFcn',gcbh);  PreSaveFcn=sps_rtmsupport('PreSaveFcn',gcbh);  PostSaveFcn=sps_rtmsupport('PostSaveFcn',gcbh);  PreCopyFcn=sps_rtmsupport('PreCopyFcn',gcbh);  OpenFcn=sps_rtmsupport('OpenFcn',gcbh, [1 -2]);  CloseFcn=sps_rtmsupport('CloseFcn',gcbh);  PreDeleteFcn=sps_rtmsupport('PreDeleteFcn',gcbh);
      settings: NameChangeFcn=|
      | sps_rtmsupport('NameChangeFcn',gcbh);
      | powericon('SetNewGotoTag',[gcb,'/source'],-2);
      mask Help: helpview(psbhelp);
      mask TypeOptions OutputType: Complex | Real-Imag | Magnitude-Angle | Magnitude
  Current Measurement2 : Subsystem  DialogController=POWERSYS.PowerSysDialog  LoadFcn=sps_rtmsupport('LoadFcn',gcbh);  StartFcn=sps_rtmsupport('StartFcn',gcbh);  StopFcn=sps_rtmsupport('StopFcn',gcbh);  mask(Current Measurement){PhasorSimulation=off, OutputType=Complex, PSBequivalent=0}
      mask prompts: PhasorSimulation "Phasor simulation"; OutputType "Output signal :"; PSBequivalent "Equivalent circuit"
      mask help: Ideal current measurement. The Output signal parameter is disabled when the block is not used in a phasor simulation. The phasor simulation is activated by a Powergui block placed in the model.
      mask init: same as myLibrary/HVDC_line/Current Measurement1
      settings: LibrarySourceBlock=sps_lib/Sensors and Measurements/Current Measurement  CopyFcn=sps_rtmsupport('CopyFcn',gcbh); powericon('psbloadfunction',gcb,'Measurement Block','UpdateGotoTag');  DeleteFcn=sps_rtmsupport('DeleteFcn',gcbh);  UndoDeleteFcn=sps_rtmsupport('UndoDeleteFcn',gcbh);  ModelCloseFcn=sps_rtmsupport('ModelCloseFcn',gcbh);  PreSaveFcn=sps_rtmsupport('PreSaveFcn',gcbh);  PostSaveFcn=sps_rtmsupport('PostSaveFcn',gcbh);  PreCopyFcn=sps_rtmsupport('PreCopyFcn',gcbh);  OpenFcn=sps_rtmsupport('OpenFcn',gcbh, [1 -2]);  CloseFcn=sps_rtmsupport('CloseFcn',gcbh);  PreDeleteFcn=sps_rtmsupport('PreDeleteFcn',gcbh);
      settings: NameChangeFcn=|
      | sps_rtmsupport('NameChangeFcn',gcbh);
      | powericon('SetNewGotoTag',[gcb,'/source'],-2);
      mask Help: helpview(psbhelp);
      mask TypeOptions OutputType: Complex | Real-Imag | Magnitude-Angle | Magnitude
  Demux : Demux  Outputs=3
  Demux1 : Demux  Outputs=3
  Demux2 : Demux  Outputs=2
  Mux : Mux  Inputs=3
  Mux1 : Mux  Inputs=3
  Mux10 : Mux  Inputs=2
  ParkInverse : Subsystem  mask(Gerard){}
      mask help:
      | This block applies the park inverse transfomation from a desired vector.
      | The input Xqd0 refers to the vector in the qd0 frame, and the second input is the angle used in the inverse transformation.
      | The output is the vector in the ABC frame.
      mask Display:
      | port_label('output',1,'Xabc')
      | port_label('input',1,'Xqd0')
      | port_label('input',2,'angle')
  ParkTransform10 : Subsystem  mask(Gerard){}
      mask help:
      | This block applies the park transfomation from a desired vector.
      | The input Xabc refers to the vector in the ABC frame, and the second input is the angle used in the transformation.
      | The output is the vector in the qd0 frame.
      mask Display:
      | port_label('output',1,'Xqd0')
      | port_label('input',1,'Xabc')
      | port_label('input',2,'angle')
  Product4 : Product  Multiplication=Matrix(*)
  Scope : Scope  NumInputPorts=2
  Scope1 : Scope
  Scope2 : Scope  NumInputPorts=2
  Scope3 : Scope  NumInputPorts=3
  Series RLC Branch : spsSeriesRLCBranchLib/Series RLC Branch  LConnTagsString=__new0  RConnTagsString=__new0  BranchType=R  Resistance=T_user.Sn(num)*1000  Inductance=1e-3  SetiL0=off  InitialCurrent=0  Capacitance=1e-6  Setx0=off  InitialVoltage=0  Measurements=None
  Series RLC Branch1 : PMComponent  DialogController=POWERSYS.PowerSysDialog  LoadFcn=sps_rtmsupport('LoadFcn',gcbh);  StartFcn=sps_rtmsupport('StartFcn',gcbh);  StopFcn=sps_rtmsupport('StopFcn',gcbh);  PhysicalDomain=powersysdomain  LeftPortType=p1  RightPortType=p1  LConnTagsString=__new0  RConnTagsString=__new0  mask(Series RLC Branch){BranchType=R, Resistance=T_user.Sn(num)*1000, Inductance=1e-3, SetiL0=off, InitialCurrent=0, Capacitance=1e-6, Setx0=off, InitialVoltage=0, Measurements=None}
      mask prompts: BranchType "Branch type:"; Resistance "Resistance (Ohms):"; Inductance "Inductance (H):"; SetiL0 "Set the initial inductor current"; InitialCurrent "Inductor initial current (A):"; Capacitance "Capacitance (F):"; Setx0 "Set the initial capacitor voltage"; InitialVoltage "Capacitor initial voltage (V):"
      mask help:
      | Implements a series branch of RLC elements.
      | Use the 'Branch type' parameter to add or remove elements from the branch.
      mask init:
      | [s1,s2,s3,s4,r1,r2,l1,l2,c1,c2,c3,c4] = powericon('Series RLC Branch',Resistance,Inductance,Capacitance,BranchType);
      | powericon('RLCCback',gcb)
      | power_initmask();
      settings: LibrarySourceBlock=sps_lib/Passives/Series RLC Branch  CopyFcn=sps_rtmsupport('CopyFcn',gcbh);  DeleteFcn=sps_rtmsupport('DeleteFcn',gcbh);  UndoDeleteFcn=sps_rtmsupport('UndoDeleteFcn',gcbh);  ModelCloseFcn=sps_rtmsupport('ModelCloseFcn',gcbh);  PreSaveFcn=sps_rtmsupport('PreSaveFcn',gcbh);  PostSaveFcn=sps_rtmsupport('PostSaveFcn',gcbh);  NameChangeFcn=sps_rtmsupport('NameChangeFcn',gcbh);  PreCopyFcn=sps_rtmsupport('PreCopyFcn',gcbh);  OpenFcn=sps_rtmsupport('OpenFcn',gcbh, [1 4 7 9]);  CloseFcn=sps_rtmsupport('CloseFcn',gcbh);  PreDeleteFcn=sps_rtmsupport('PreDeleteFcn',gcbh);
      mask Help: helpview(psbhelp);
      mask TypeOptions BranchType: RLC | R | L | C | RL | RC | LC | Open circuit
      mask Callback BranchType: powericon('RLCCback',gcb)
      mask Callback Resistance: powericon('RLCCback',gcb)
      mask Callback Inductance: powericon('RLCCback',gcb)
      mask Callback SetiL0: powericon('RLCCback',gcb)
      mask Callback Capacitance: powericon('RLCCback',gcb)
      mask Callback Setx0: powericon('RLCCback',gcb)
      mask TypeOptions Measurements: None | Branch voltage | Branch current | Branch voltage and current
      mask Display:
      | plot(s1,s2,s3,s4,r1,r2*1.5,l1,l2*1.5,c1,c2*1.5,c3,c4*1.5)
      | color('red')
      | port_label('LConn',1,'+')
  Series RLC Branch2 : PMComponent  DialogController=POWERSYS.PowerSysDialog  LoadFcn=sps_rtmsupport('LoadFcn',gcbh);  StartFcn=sps_rtmsupport('StartFcn',gcbh);  StopFcn=sps_rtmsupport('StopFcn',gcbh);  PhysicalDomain=powersysdomain  LeftPortType=p1  RightPortType=p1  LConnTagsString=__new0  RConnTagsString=__new0  mask(Series RLC Branch){BranchType=R, Resistance=T_user.Sn(num)*1000, Inductance=1e-3, SetiL0=off, InitialCurrent=0, Capacitance=1e-6, Setx0=off, InitialVoltage=0, Measurements=None}
      mask prompts: BranchType "Branch type:"; Resistance "Resistance (Ohms):"; Inductance "Inductance (H):"; SetiL0 "Set the initial inductor current"; InitialCurrent "Inductor initial current (A):"; Capacitance "Capacitance (F):"; Setx0 "Set the initial capacitor voltage"; InitialVoltage "Capacitor initial voltage (V):"
      mask help:
      | Implements a series branch of RLC elements.
      | Use the 'Branch type' parameter to add or remove elements from the branch.
      mask init:
      | [s1,s2,s3,s4,r1,r2,l1,l2,c1,c2,c3,c4] = powericon('Series RLC Branch',Resistance,Inductance,Capacitance,BranchType);
      | powericon('RLCCback',gcb)
      | power_initmask();
      settings: LibrarySourceBlock=sps_lib/Passives/Series RLC Branch  CopyFcn=sps_rtmsupport('CopyFcn',gcbh);  DeleteFcn=sps_rtmsupport('DeleteFcn',gcbh);  UndoDeleteFcn=sps_rtmsupport('UndoDeleteFcn',gcbh);  ModelCloseFcn=sps_rtmsupport('ModelCloseFcn',gcbh);  PreSaveFcn=sps_rtmsupport('PreSaveFcn',gcbh);  PostSaveFcn=sps_rtmsupport('PostSaveFcn',gcbh);  NameChangeFcn=sps_rtmsupport('NameChangeFcn',gcbh);  PreCopyFcn=sps_rtmsupport('PreCopyFcn',gcbh);  OpenFcn=sps_rtmsupport('OpenFcn',gcbh, [1 4 7 9]);  CloseFcn=sps_rtmsupport('CloseFcn',gcbh);  PreDeleteFcn=sps_rtmsupport('PreDeleteFcn',gcbh);
      mask Help: helpview(psbhelp);
      mask TypeOptions BranchType: RLC | R | L | C | RL | RC | LC | Open circuit
      mask Callback BranchType: powericon('RLCCback',gcb)
      mask Callback Resistance: powericon('RLCCback',gcb)
      mask Callback Inductance: powericon('RLCCback',gcb)
      mask Callback SetiL0: powericon('RLCCback',gcb)
      mask Callback Capacitance: powericon('RLCCback',gcb)
      mask Callback Setx0: powericon('RLCCback',gcb)
      mask TypeOptions Measurements: None | Branch voltage | Branch current | Branch voltage and current
      mask Display:
      | plot(s1,s2,s3,s4,r1,r2*1.5,l1,l2*1.5,c1,c2*1.5,c3,c4*1.5)
      | color('red')
      | port_label('LConn',1,'+')
  State-Space : StateSpace  A=T_user.A{num}  B=T_user.B{num}  C=T_user.C{num}  D=T_user.D{num}  InitialCondition=0
  Sum : Sum  Inputs=++|
  Sum1 : Sum  Inputs=|++
  Sum2 : Sum  Inputs=-+|
  Sum3 : Sum  Inputs=|+-
  Sum7 : Sum  Inputs=|+-
  Terminator : Terminator
  Terminator1 : Terminator
  Unit Delay1 : UnitDelay  Commented=on  InitialCondition=inituser.vg_q0  SampleTime=1e-5  HasFrameUpgradeWarning=on
  Unit Delay4 : UnitDelay  Commented=on  InitialCondition=inituser.vg_d0  SampleTime=1e-5  HasFrameUpgradeWarning=on
  Voltage Measurement : Subsystem  DialogController=POWERSYS.PowerSysDialog  LoadFcn=sps_rtmsupport('LoadFcn',gcbh);  StartFcn=sps_rtmsupport('StartFcn',gcbh);  StopFcn=sps_rtmsupport('StopFcn',gcbh);  mask(Voltage Measurement){PhasorSimulation=off, OutputType=Complex, PSBequivalent=0}
      mask prompts: PhasorSimulation "Phasor simulation"; OutputType "Output signal :"; PSBequivalent "Equivalent circuit"
      mask help: Ideal voltage measurement. The Output signal parameter is disabled when the block is not used in a phasor simulation. The phasor simulation is activated by a Powergui block placed in the model.
      mask init: same as myLibrary/HVDC_line/Current Measurement1
      settings: LibrarySourceBlock=sps_lib/Sensors and Measurements/Voltage Measurement  CopyFcn=sps_rtmsupport('CopyFcn',gcbh); powericon('psbloadfunction',gcb,'Measurement Block','UpdateGotoTag');  DeleteFcn=sps_rtmsupport('DeleteFcn',gcbh);  UndoDeleteFcn=sps_rtmsupport('UndoDeleteFcn',gcbh);  ModelCloseFcn=sps_rtmsupport('ModelCloseFcn',gcbh);  PreSaveFcn=sps_rtmsupport('PreSaveFcn',gcbh);  PostSaveFcn=sps_rtmsupport('PostSaveFcn',gcbh);  NameChangeFcn=sps_rtmsupport('NameChangeFcn',gcbh);powericon('SetNewGotoTag',[gcb,'/source'],-2);  PreCopyFcn=sps_rtmsupport('PreCopyFcn',gcbh);  OpenFcn=sps_rtmsupport('OpenFcn',gcbh, [1 -2]);  CloseFcn=sps_rtmsupport('CloseFcn',gcbh);  PreDeleteFcn=sps_rtmsupport('PreDeleteFcn',gcbh);
      mask Help: helpview(psbhelp);
      mask TypeOptions OutputType: Complex | Real-Imag | Magnitude-Angle | Magnitude
  Voltage Measurement1 : Subsystem  DialogController=POWERSYS.PowerSysDialog  LoadFcn=sps_rtmsupport('LoadFcn',gcbh);  StartFcn=sps_rtmsupport('StartFcn',gcbh);  StopFcn=sps_rtmsupport('StopFcn',gcbh);  mask(Voltage Measurement){PhasorSimulation=off, OutputType=Complex, PSBequivalent=0}
      mask prompts: PhasorSimulation "Phasor simulation"; OutputType "Output signal :"; PSBequivalent "Equivalent circuit"
      mask help: Ideal voltage measurement. The Output signal parameter is disabled when the block is not used in a phasor simulation. The phasor simulation is activated by a Powergui block placed in the model.
      mask init: same as myLibrary/HVDC_line/Current Measurement1
      settings: LibrarySourceBlock=sps_lib/Sensors and Measurements/Voltage Measurement  CopyFcn=sps_rtmsupport('CopyFcn',gcbh); powericon('psbloadfunction',gcb,'Measurement Block','UpdateGotoTag');  DeleteFcn=sps_rtmsupport('DeleteFcn',gcbh);  UndoDeleteFcn=sps_rtmsupport('UndoDeleteFcn',gcbh);  ModelCloseFcn=sps_rtmsupport('ModelCloseFcn',gcbh);  PreSaveFcn=sps_rtmsupport('PreSaveFcn',gcbh);  PostSaveFcn=sps_rtmsupport('PostSaveFcn',gcbh);  NameChangeFcn=sps_rtmsupport('NameChangeFcn',gcbh);powericon('SetNewGotoTag',[gcb,'/source'],-2);  PreCopyFcn=sps_rtmsupport('PreCopyFcn',gcbh);  OpenFcn=sps_rtmsupport('OpenFcn',gcbh, [1 -2]);  CloseFcn=sps_rtmsupport('CloseFcn',gcbh);  PreDeleteFcn=sps_rtmsupport('PreDeleteFcn',gcbh);
      mask Help: helpview(psbhelp);
      mask TypeOptions OutputType: Complex | Real-Imag | Magnitude-Angle | Magnitude
  A : PMIOPort  Side=Right
  B : PMIOPort  Port=2  Side=Right
  C : PMIOPort  Port=3  Side=Right
  wires:
  Demux/1 -> Controlled Current Source/1, Scope/1
  Mux/1 -> State-Space/1
  ParkTransform10/1(qd0 vector) -> Demux1/1
  Demux1/3 -> Terminator/1
  ParkInverse/1(Matrix) -> Demux/1
  Demux/3 -> Terminator1/1
  Constant5/1 -> Product4/1
  Mux10/1 -> Product4/2
  Product4/1 -> Scope1/1, ParkTransform10/1(ABC vector)
  Voltage Measurement/1(v) -> Mux10/1
  Voltage Measurement1/1(v) -> Mux10/2
  Constant/1 -> Mux1/3
  Demux2/1 -> Sum/2
  Demux2/2 -> Sum1/1
  Constant1/1 -> Sum/1
  Constant2/1 -> Sum1/2
  Sum2/1 -> Mux/1
  Demux1/1 -> Sum2/2, Scope2/1  "Vq"
  Sum3/1 -> Mux/2
  Demux1/2 -> Scope2/2, Sum3/1  "Vd"
  Constant3/1 -> Sum2/1
  Constant4/1 -> Sum3/2
  State-Space/1 -> Demux2/1
  Mux1/1 -> ParkInverse/1(ABC vector)
  Sum/1 -> Mux1/1
  Sum1/1 -> Mux1/2
  [angle_ref1] -> ParkInverse/2(angle), ParkTransform10/2(angle)
  [w_TH38] -> Sum7/1
  Constant8/1 -> Sum7/2
  Sum7/1 -> Mux/3
  Demux/2 -> Scope/2, Controlled Current Source1/1
  Current Measurement/1 -> Scope3/1
  Current Measurement1/1(i) -> Scope3/2
  Current Measurement2/1(i) -> Scope3/3
  connections:
  Voltage Measurement/LConn1 -- Current Measurement/LConn1 -- Controlled Current Source/RConn1 -- A/RConn1
  Controlled Current Source/LConn1 -- Current Measurement2/LConn1 -- Voltage Measurement1/LConn2 -- C/RConn1 -- Controlled Current Source1/LConn1
  Voltage Measurement1/LConn1 -- Current Measurement1/LConn1 -- Controlled Current Source1/RConn1 -- Voltage Measurement/LConn2 -- B/RConn1
  Series RLC Branch/RConn1 -- Series RLC Branch1/RConn1 -- Series RLC Branch2/RConn1
  Current Measurement/RConn1 -- Series RLC Branch/LConn1
  Current Measurement2/RConn1 -- Series RLC Branch2/LConn1
  Current Measurement1/RConn1 -- Series RLC Branch1/LConn1

== system myLibrary/User-Non-Linear ==
  note: Paste the non-linear model
  Constant : Constant  Value=0
  Constant1 : Constant  Value=init_user{num}.ig_qc0_nl
  Constant2 : Constant  Value=init_user{num}.ig_dc0_nl
  Constant3 : Constant  Value=0
  Constant4 : Constant  Value=2*pi*T_user.fn(num)
  Constant5 : Constant  Value=[ 2/3 1/3; -1/3 1/3 ; -1/3 -2/3]
  Controlled Current Source : spsControlledCurrentSourceLib/Controlled Current Source  Initialize=on  Source_Type=AC  Amplitude=abs(init_user{num}.Igabc_nl)*sqrt(2)  Phase=init_user{num}.angle_Ig*180/pi  Frequency=T_user.fn(num)  Measurements=None
  Controlled Current Source1 : spsControlledCurrentSourceLib/Controlled Current Source  Initialize=on  Source_Type=AC  Amplitude=abs(init_user{num}.Igabc_nl)*sqrt(2)  Phase=init_user{num}.angle_Ig*180/pi+120  Frequency=T_user.fn(num)  Measurements=None
  Current Measurement : spsCurrentMeasurementLib/Current Measurement  PhasorSimulation=off  OutputType=Complex  PSBequivalent=0
  Current Measurement1 : Subsystem  DialogController=POWERSYS.PowerSysDialog  LoadFcn=sps_rtmsupport('LoadFcn',gcbh);  StartFcn=sps_rtmsupport('StartFcn',gcbh);  StopFcn=sps_rtmsupport('StopFcn',gcbh);  mask(Current Measurement){PhasorSimulation=off, OutputType=Complex, PSBequivalent=0}
      mask prompts: PhasorSimulation "Phasor simulation"; OutputType "Output signal :"; PSBequivalent "Equivalent circuit"
      mask help: Ideal current measurement. The Output signal parameter is disabled when the block is not used in a phasor simulation. The phasor simulation is activated by a Powergui block placed in the model.
      mask init: same as myLibrary/HVDC_line/Current Measurement1
      settings: LibrarySourceBlock=sps_lib/Sensors and Measurements/Current Measurement  CopyFcn=sps_rtmsupport('CopyFcn',gcbh); powericon('psbloadfunction',gcb,'Measurement Block','UpdateGotoTag');  DeleteFcn=sps_rtmsupport('DeleteFcn',gcbh);  UndoDeleteFcn=sps_rtmsupport('UndoDeleteFcn',gcbh);  ModelCloseFcn=sps_rtmsupport('ModelCloseFcn',gcbh);  PreSaveFcn=sps_rtmsupport('PreSaveFcn',gcbh);  PostSaveFcn=sps_rtmsupport('PostSaveFcn',gcbh);  PreCopyFcn=sps_rtmsupport('PreCopyFcn',gcbh);  OpenFcn=sps_rtmsupport('OpenFcn',gcbh, [1 -2]);  CloseFcn=sps_rtmsupport('CloseFcn',gcbh);  PreDeleteFcn=sps_rtmsupport('PreDeleteFcn',gcbh);
      settings: NameChangeFcn=|
      | sps_rtmsupport('NameChangeFcn',gcbh);
      | powericon('SetNewGotoTag',[gcb,'/source'],-2);
      mask Help: helpview(psbhelp);
      mask TypeOptions OutputType: Complex | Real-Imag | Magnitude-Angle | Magnitude
  Current Measurement2 : Subsystem  DialogController=POWERSYS.PowerSysDialog  LoadFcn=sps_rtmsupport('LoadFcn',gcbh);  StartFcn=sps_rtmsupport('StartFcn',gcbh);  StopFcn=sps_rtmsupport('StopFcn',gcbh);  mask(Current Measurement){PhasorSimulation=off, OutputType=Complex, PSBequivalent=0}
      mask prompts: PhasorSimulation "Phasor simulation"; OutputType "Output signal :"; PSBequivalent "Equivalent circuit"
      mask help: Ideal current measurement. The Output signal parameter is disabled when the block is not used in a phasor simulation. The phasor simulation is activated by a Powergui block placed in the model.
      mask init: same as myLibrary/HVDC_line/Current Measurement1
      settings: LibrarySourceBlock=sps_lib/Sensors and Measurements/Current Measurement  CopyFcn=sps_rtmsupport('CopyFcn',gcbh); powericon('psbloadfunction',gcb,'Measurement Block','UpdateGotoTag');  DeleteFcn=sps_rtmsupport('DeleteFcn',gcbh);  UndoDeleteFcn=sps_rtmsupport('UndoDeleteFcn',gcbh);  ModelCloseFcn=sps_rtmsupport('ModelCloseFcn',gcbh);  PreSaveFcn=sps_rtmsupport('PreSaveFcn',gcbh);  PostSaveFcn=sps_rtmsupport('PostSaveFcn',gcbh);  PreCopyFcn=sps_rtmsupport('PreCopyFcn',gcbh);  OpenFcn=sps_rtmsupport('OpenFcn',gcbh, [1 -2]);  CloseFcn=sps_rtmsupport('CloseFcn',gcbh);  PreDeleteFcn=sps_rtmsupport('PreDeleteFcn',gcbh);
      settings: NameChangeFcn=|
      | sps_rtmsupport('NameChangeFcn',gcbh);
      | powericon('SetNewGotoTag',[gcb,'/source'],-2);
      mask Help: helpview(psbhelp);
      mask TypeOptions OutputType: Complex | Real-Imag | Magnitude-Angle | Magnitude
  Demux : Demux  Outputs=3
  Demux1 : Demux  Outputs=3
  Integrator1 : Integrator
  Integrator2 : Integrator  InitialCondition=init_user{num}.angles_nl
  Ki : Gain  Gain=T_user.ki_pll(num)
  Kp : Gain  Gain=T_user.kp_pll(num)
  Mux : Mux  Inputs=3
  Mux10 : Mux  Inputs=2
  ParkInverse : $bdroot/User-Linear/ParkInverse
  ParkTransform10 : $bdroot/User-Linear/ParkTransform10
  Product4 : Product  Multiplication=Matrix(*)
  Scope{,1..4,6} (6 alike) : Scope
  Scope5 : Scope  NumInputPorts=3
  Sum : Sum  Inputs=|-+
  Sum1 : Sum  Inputs=|++
  Sum2 : Sum  Inputs=|++
  Terminator : Terminator
  Terminator1 : Terminator
  Terminator2 : Terminator
  Voltage Measurement : $bdroot/User-Linear/Voltage Measurement  PhasorSimulation=off  OutputType=Complex  PSBequivalent=0
      settings: LibrarySourceBlock=sps_lib/Sensors and Measurements/Voltage Measurement
  Voltage Measurement1 : $bdroot/User-Linear/Voltage Measurement1  PhasorSimulation=off  OutputType=Complex  PSBequivalent=0
      settings: LibrarySourceBlock=sps_lib/Sensors and Measurements/Voltage Measurement
  A : PMIOPort  Side=Right
  B : PMIOPort  Port=2  Side=Right
  C : PMIOPort  Port=3  Side=Right
  wires:
  Demux/2 -> Controlled Current Source1/1
  Demux/1 -> Controlled Current Source/1
  ParkInverse/1 -> Scope/1, Demux/1
  Voltage Measurement1/1 -> Mux10/2
  Product4/1 -> Scope6/1, ParkTransform10/1
  Demux/3 -> Terminator1/1
  Constant5/1 -> Product4/1
  Voltage Measurement/1 -> Mux10/1
  Mux10/1 -> Product4/2
  Ki/1 -> Integrator1/1
  Constant/1 -> Sum/2
  Kp/1 -> Sum1/1
  Integrator1/1 -> Sum1/2
  Sum/1 -> Kp/1, Ki/1
  ParkTransform10/1 -> Scope4/1, Demux1/1
  Demux1/2 -> Scope3/1, Sum/1
  Demux1/1 -> Terminator/1
  Demux1/3 -> Terminator2/1
  Mux/1 -> ParkInverse/1
  Constant1/1 -> Mux/1
  Constant2/1 -> Mux/2
  Constant3/1 -> Mux/3
  Integrator2/1 -> ParkInverse/2, Scope1/1, ParkTransform10/2
  Sum2/1 -> Scope2/1, Integrator2/1
  Sum1/1 -> Sum2/1
  Constant4/1 -> Sum2/2
  Current Measurement2/1(i) -> Scope5/1
  Current Measurement/1 -> Scope5/2
  Current Measurement1/1(i) -> Scope5/3
  connections:
  Controlled Current Source/LConn1 -- Current Measurement1/LConn1 -- Controlled Current Source1/LConn1
  B/RConn1 -- Current Measurement/RConn1 -- Voltage Measurement/LConn2 -- Voltage Measurement1/LConn1
  Voltage Measurement/LConn1 -- A/RConn1 -- Current Measurement2/RConn1
  C/RConn1 -- Current Measurement1/RConn1 -- Voltage Measurement1/LConn2
  Current Measurement/LConn1 -- Controlled Current Source1/RConn1
  Current Measurement2/LConn1 -- Controlled Current Source/RConn1
